simulink model "NonlinearSim"  (R2020a)
settings: Solver=ode45  StartTime=0.0  StopTime=20  FixedStep=1e-3  RelTol=1e-3  EnableMultiTasking=on
values from neighbouring files (symbols this model uses):
  b = 0.05    [Main.m]
  m = 0.25    [Main.m]
  M = 1.0    (= 1)    [Main.m]
libraries: cstblocks x1, simulink x1
settings Model: Creator=FawaD KhaN  LastModifiedBy=FawaD KhaN
settings DataIOCC: LimitDataPoints=on  SaveFormat=Array  ReturnWorkspaceOutputs=off
settings OptimizationCC: LifeSpan=inf
settings DebuggingCC: SFUnexpectedBacktrackingDiag=warning  SFNoUnconditionalDefaultTransitionDiag=warning  SFExecutionAtInitializationDiag=none  ArithmeticOperatorsInVariantConditions=warning
settings HardwareCC: ProdBitPerPointer=32  ProdBitPerSizeT=32  ProdBitPerPtrDiffT=32  ProdLargestAtomicFloat=None  ProdIntDivRoundTo=Undefined  ProdEndianess=Unspecified  ProdWordSize=32  ProdHWDeviceType=32-bit Generic
settings ModelReferenceCC: PropagateSignalLabelsOutOfModel=off
settings SFSimCC: SimUseLocalCustomCode=off  CustomCodeUndefinedFunction=UseInterfaceOnly
settings RTWCC: RTWUseLocalCustomCode=off
settings CodeAppCC: StateflowObjectComments=on
settings GRTTargetCC: TargetLangStandard=C89/C90 (ANSI)
settings ConfigComp: CovMetricSettings=dw  CovHtmlReporting=on  CovSaveCumulativeToWorkspaceVar=on  CovSaveSingleToWorkspaceVar=on  CovExternalEMLEnable=off

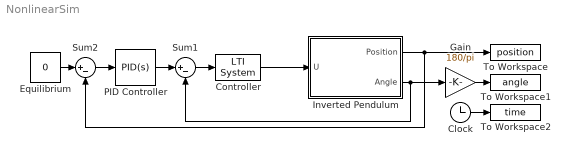
== system NonlinearSim ==
  Clock : Clock
  Controller : cstblocks/LTI System  sys=K  IC=[]
  Equilibrium : Constant  Value=0
  Gain : Gain  Gain=180/pi
  Inverted Pendulum : Subsystem
  PID Controller : simulink/Continuous/PID Controller  Controller=PID  Form=Parallel  TimeDomain=Continuous-time  UseExternalTs=off  SampleTime=-1  IntegratorMethod=Forward Euler  FilterMethod=Forward Euler  ControllerParametersSource=internal  P=0.0193530389363055  I=0.000993819105270644  D=0.0759239973431993  UseFilter=on  N=5.15691532233635  TunerSelectOption=Transfer Function Based (PID Tuner App)  InitialConditionSource=internal  InitialConditionForIntegrator=0  InitialConditionForFilter=0  DifferentiatorICPrevScaledInput=0  ExternalReset=none  TrackingMode=off  Kt=1  LimitOutput=off  UpperSaturationLimit=inf  LowerSaturationLimit=-inf  LinearizeAsGain=on  AntiWindupMode=none  Kb=1  POutMin=[]  POutMax=[]  IOutMin=[]  IOutMax=[]  DOutMin=[]  DOutMax=[]  NOutMin=[]  NOutMax=[]  SumOutMin=[]  SumOutMax=[]  SaturationOutMin=[]  SaturationOutMax=[]  PParamMin=[]  PParamMax=[]  IParamMin=[]  IParamMax=[]  DParamMin=[]  DParamMax=[]  NParamMin=[]  NParamMax=[]  KbParamMin=[]  KbParamMax=[]  KtParamMin=[]  KtParamMax=[]  KbOutMin=[]  KbOutMax=[]  KtOutMin=[]  KtOutMax=[]  IntegratorOutMin=[]  IntegratorOutMax=[]  FilterOutMin=[]  FilterOutMax=[]  SumI1OutMin=[]  SumI1OutMax=[]  SumI2OutMin=[]  SumI2OutMax=[]  SumI3OutMin=[]  SumI3OutMax=[]  SumI4OutMin=[]  SumI4OutMax=[]  SumDOutMin=[]  SumDOutMax=[]  DifferentiatorOutMin=[]  DifferentiatorOutMax=[]  FilterDiffOutCoefMin=[]  FilterDiffOutCoefMax=[]  ReciprocalOutMin=[]  ReciprocalOutMax=[]  SumDenOutMin=[]  SumDenOutMax=[]  SumNumOutMin=[]  SumNumOutMax=[]  DivideOutMin=[]  DivideOutMax=[]  UdiffTsProdOutMin=[]  UdiffTsProdOutMax=[]  NTsProdOutMin=[]  NTsProdOutMax=[]  UintegralTsProdOutMin=[]  UintegralTsProdOutMax=[]  UngainTsProdOutMin=[]  UngainTsProdOutMax=[]  IntegratorContinuousStateAttributes=''  IntegratorStateMustResolveToSignalObject=off  IntegratorRTWStateStorageClass=Auto  FilterContinuousStateAttributes=''  FilterStateMustResolveToSignalObject=off  FilterRTWStateStorageClass=Auto  ParallelPVariant=InternalParameters  IdealPVariant=Disabled  IVariant=InternalParameters  DVariant=InternalParameters  IntegratorVariant=Continuous  SatVariant=Disabled  AWVariant=Passthrough  PCopyVariant=Disabled  TRVariant=Disabled  FdbkBlocksVariant=Forward  IdealPFdbkVariant=Disabled  SatFdbkVariant=Disabled  DerivativeFilterVariant=ContFilter  NVariant=InternalParameters  NCopyVariant=Disabled  FilterICVariant=InternalICsFilter  IntegratorICVariant=InternalICs  ExternalResetVariant=Disabled  TRSumVariant=Passthrough  SumFdbkVariant=Disabled  SumVariant=Sum_PID  TsampFilterVariant=InternalTs  TsampNgainVariant=Passthrough  TsampIntegralVariant=Passthrough
  Sum1 : Sum  Inputs=|+-
  Sum2 : Sum  Inputs=|+-
  To Workspace : ToWorkspace  VariableName=position  SampleTime=-1
  To Workspace1 : ToWorkspace  VariableName=angle  SampleTime=-1
  To Workspace2 : ToWorkspace  VariableName=time  SampleTime=-1
  wires:
  Gain/1 -> To Workspace1/1
  Sum1/1 -> Controller/1
  PID Controller/1 -> Sum1/1
  Sum2/1 -> PID Controller/1
  Equilibrium/1 -> Sum2/1
  Controller/1 -> Inverted Pendulum/1(U)
  Clock/1 -> To Workspace2/1
  Inverted Pendulum/2(Angle) -> Gain/1, Sum1/2
  Inverted Pendulum/1(Position) -> To Workspace/1, Sum2/2

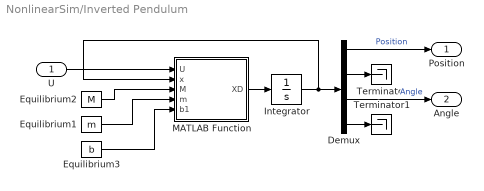
== system NonlinearSim/Inverted Pendulum ==
  U : Inport
  Demux : Demux
  Equilibrium1 : Constant  Value=m
  Equilibrium2 : Constant  Value=M
  Equilibrium3 : Constant  Value=b
  Integrator : Integrator  InitialCondition=[0;0;pi/3;0]
  MATLAB Function : MATLAB Function  TreatAsAtomicUnit=on
  Terminator : Terminator
  Terminator1 : Terminator
  Position : Outport
  Angle : Outport  Port=2
  wires:
  Equilibrium2/1 -> MATLAB Function/3(M)
  MATLAB Function/1(XD) -> Integrator/1
  U/1 -> MATLAB Function/1(U)
  Equilibrium1/1 -> MATLAB Function/4(m)
  Demux/3 -> Angle/1  "Angle"
  Demux/1 -> Position/1  "Position"
  Demux/2 -> Terminator/1
  Demux/4 -> Terminator1/1
  Integrator/1 -> Demux/1, MATLAB Function/2(x)
  Equilibrium3/1 -> MATLAB Function/5(b1)

== matlab function NonlinearSim/Inverted Pendulum/MATLAB Function ==
  data: U input; XD output; x input; M input; m input; b1 input
function XD = fcn(U,x,M,m,b1)
l  = 0.5;
b1 = 0.05;
g  = 9.81;

%% assign states
y  = x(1);
dy = x(2);
theta  = x(3);
dtheta = x(4);

%% assign inputs
F = U(1);
%% Compute Derivatives
ydot     = dy;
thetadot = dtheta;

M = [M+m, m*(l/2)*cos(theta);...
     m*(l/2)*cos(theta), m*(l^2)/4];
 
c = [m*(l/2)*thetadot^2*sin(theta) + F - b1*ydot;...
     m*g*(l/2)*sin(theta)];
 
tmp = M\c;

yddot = tmp(1);
thetaddot = tmp(2);
n = [ydot;yddot];
q = [thetadot;thetaddot];

XD = [n;q];
